simulink model "SPMSM_Speed_Control"  (R2023b)
settings: Solver=ode45  StartTime=0.0  StopTime=10  MaxStep=0.001  RelTol=1e-3
values from neighbouring files (symbols this model uses):
  J_motor = 0.0027    [PMSM_parameter2.m]
  Lamda = 0.1194    [PMSM_parameter2.m]
  Ld = 0.0003752    [PMSM_parameter2.m]
  Lq = 0.0003752    [PMSM_parameter2.m]
  Pole = 2    [PMSM_parameter2.m]
  R = 0.2    [PMSM_parameter2.m]
  T_load = 10    [PMSM_parameter2.m]
  w_base = (60/(2*pi))*(v_rated/sqrt((Ls^2)*(T_load/1.5*Pole*Lamda)^2+(Lamda^2)))    [PMSM_parameter2.m]
  w_ref = 3000    [PMSM_parameter2.m]
undefined symbols (not defined in the file or in its folder): v_rated
libraries: mcbcontrolslib x10, slpidlib x6, autolibpmsmexterior x2, simulink_extras x1, autolibpmsmcommon x1, spsSawtoothGeneratorLib x1
settings Model: Creator=chayutht  LastModifiedBy=chayutht
settings DebuggingCC: AlgebraicLoopMsg=none  ArtificialAlgebraicLoopMsg=none

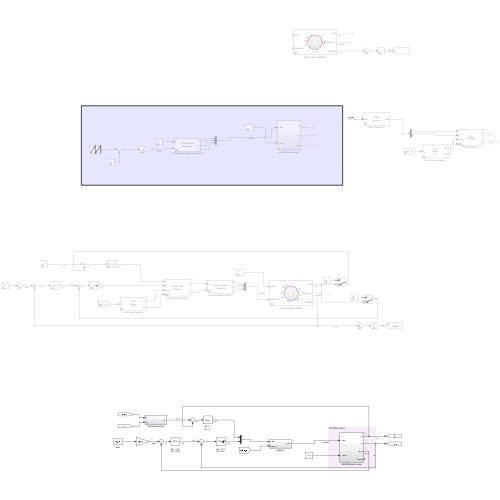
[thumbnail: Simulink's stored preview of the top-level diagram]
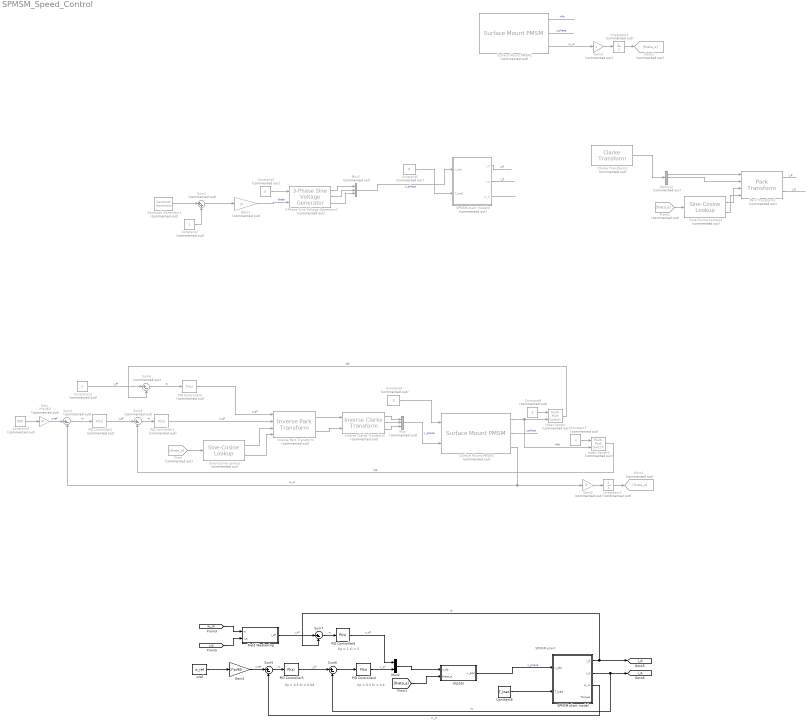
== system SPMSM_Speed_Control ==
  note: SPMSM plant
  note: Kp = 1
      | Ki = 5
  note: Kp = 0.3
      | Ki = 0.4
  note: Kp = 0.5
      | Ki = 0.08
  3-Phase Sine Voltage Generator2 : mcbcontrolslib/3-Phase Sine Voltage Generator  Commented=on  AngleInput=Radians  N_points=1024
      settings: LibrarySourceBlock=mcblib/Controls/Math Transforms/3-Phase Sine Voltage Generator
  Clarke Transform1 : mcbcontrolslib/Clarke Transform  Commented=on  VariantControl=Variant2  PhaseInput=Three inputs  EnPowerInv=off
      settings: LibrarySourceBlock=mcblib/Controls/Math Transforms/Clarke Transform
  Constant10 : Constant  Commented=on  Value=0
  Constant2 : Constant  Commented=on
  Constant3 : Constant  Commented=on  Value=5
  Constant4 : Constant  Commented=on  Value=0
  Constant5 : Constant  Commented=on  Value=0
  Constant6 : Constant  Commented=on  Value=3
  Constant7 : Constant  Commented=on  Value=4
  Constant8 : Constant  Value=T_load
  Constant9 : Constant  Commented=on  Value=500
  Demux2 : Demux  Commented=on  Outputs=3
  Field Weakening : Subsystem
  From : From  Commented=on  GotoTag=theta_e
  From2 : From  Commented=on  GotoTag=theta_e
  Gain : Gain  Commented=on  Gain=2*pi/60
  Gain1 : Gain  Commented=on  Gain=pi
  Gain2 : Gain  Commented=on  Gain=2
  Gain3 : Gain  Commented=on  Gain=2
  Gain4 : Gain  Gain=2*pi/60
  Goto1 : Goto  Commented=on  GotoTag=theta_e
  Goto2 : Goto  Commented=on  GotoTag=theta_e
  Index Vector : MultiPortSwitch  Commented=on  DataPortOrder=Zero-based contiguous  Inputs=1  zeroidx=on  SaturateOnIntegerOverflow=off  InputSameDT=off
  Index Vector1 : MultiPortSwitch  Commented=on  DataPortOrder=Zero-based contiguous  Inputs=1  zeroidx=on  SaturateOnIntegerOverflow=off  InputSameDT=off
  Integrator1 : Integrator  Commented=on
  Integrator2 : Integrator  Commented=on
  Inverse Clarke Transform : mcbcontrolslib/Inverse Clarke Transform  Commented=on  PhaseInput=Two inputs  EnPowerInv=off
      settings: LibrarySourceBlock=mcblib/Controls/Math Transforms/Inverse Clarke Transform
  Inverse Park Transform : mcbcontrolslib/Inverse Park Transform  Commented=on  PhaseInput=Two inputs  AxisAlignment=D-axis  ThetaInput=Sine and Cosine electrical position  AngleInput=Per-unit  N_points=1024
      settings: LibrarySourceBlock=mcblib/Controls/Math Transforms/Inverse Park Transform
  Mux : Mux  Commented=on  Inputs=3
  Mux1 : Mux  Commented=on  Inputs=3
  Mux2 : Mux  Inputs=2
  PID Controller1 : slpidlib/PID Controller  Commented=on  Controller=PI  Form=Parallel  TimeDomain=Continuous-time  UseExternalTs=off  SampleTime=-1  IntegratorMethod=Forward Euler  FilterMethod=Forward Euler  ControllerParametersSource=internal  P=3  I=1  UseKiTs=off  D=0  N=100  UseFilter=on  TunerSelectOption=Transfer Function Based (PID Tuner App)  InitialConditionSource=internal  InitialConditionForIntegrator=0  InitialConditionForFilter=0  DifferentiatorICPrevScaledInput=0  ExternalReset=none  TrackingMode=off  Kt=1  LimitOutput=on  SatLimitsSource=internal  UpperSaturationLimit=200  LowerSaturationLimit=-200  LinearizeAsGain=off  AntiWindupMode=none  Kb=1  LimitIntegrator=off  UpperIntegratorSaturationLimit=inf  LowerIntegratorSaturationLimit=-inf  POutMin=[]  POutMax=[]  IOutMin=[]  IOutMax=[]  DOutMin=[]  DOutMax=[]  NOutMin=[]  NOutMax=[]  SumOutMin=[]  SumOutMax=[]  SaturationOutMin=[]  SaturationOutMax=[]  PParamMin=[]  PParamMax=[]  IParamMin=[]  IParamMax=[]  DParamMin=[]  DParamMax=[]  NParamMin=[]  NParamMax=[]  KbParamMin=[]  KbParamMax=[]  KtParamMin=[]  KtParamMax=[]  KbOutMin=[]  KbOutMax=[]  KtOutMin=[]  KtOutMax=[]  IntegratorOutMin=[]  IntegratorOutMax=[]  FilterOutMin=[]  FilterOutMax=[]  SumI1OutMin=[]  SumI1OutMax=[]  SumI2OutMin=[]  SumI2OutMax=[]  SumI3OutMin=[]  SumI3OutMax=[]  SumI4OutMin=[]  SumI4OutMax=[]  SumDOutMin=[]  SumDOutMax=[]  DifferentiatorOutMin=[]  DifferentiatorOutMax=[]  FilterDiffOutCoefMin=[]  FilterDiffOutCoefMax=[]  ReciprocalOutMin=[]  ReciprocalOutMax=[]  SumDenOutMin=[]  SumDenOutMax=[]  SumNumOutMin=[]  SumNumOutMax=[]  DivideOutMin=[]  DivideOutMax=[]  UdiffTsProdOutMin=[]  UdiffTsProdOutMax=[]  NTsProdOutMin=[]  NTsProdOutMax=[]  UintegralTsProdOutMin=[]  UintegralTsProdOutMax=[]  UngainTsProdOutMin=[]  UngainTsProdOutMax=[]  ClampingZeroOutDataTypeStr=Inherit: Inherit via back propagation  ClampingZeroOutMin=[]  ClampingZeroOutMax=[]  FilterDenConstantOutDataTypeStr=Inherit: Inherit via back propagation  FilterDenConstantOutMin=[]  FilterDenConstantOutMax=[]  PCopyOutDataTypeStr=Inherit: Inherit via back propagation  PCopyOutMin=[]  PCopyOutMax=[]  NCopyOutDataTypeStr=Inherit: Inherit via back propagation  NCopyOutMin=[]  NCopyOutMax=[]  IntegratorContinuousStateAttributes=''  IntegratorStateMustResolveToSignalObject=off  IntegratorRTWStateStorageClass=Auto  FilterContinuousStateAttributes=''  FilterStateMustResolveToSignalObject=off  FilterRTWStateStorageClass=Auto  ParallelPVariant=InternalParameters  IdealPVariant=Disabled  IVariant=InternalParameters  DVariant=Disabled  IntegratorVariant=Continuous  SatVariant=Enabled  AWVariant=Passthrough  PCopyVariant=Disabled  TRVariant=Disabled  FdbkBlocksVariant=Forward  IdealPFdbkVariant=Disabled  SatFdbkVariant=Disabled  DerivativeFilterVariant=Disabled  NVariant=Disabled  NCopyVariant=Disabled_SignalSpec  FilterICVariant=Disabled  IntegratorICVariant=InternalICs  ExternalResetVariant=Disabled  TRSumVariant=Passthrough  SumFdbkVariant=Disabled  SumVariant=Sum_PI  TsampFilterVariant=InternalTs  TsampNgainVariant=Passthrough  TsampIntegralVariant=Disabled_SignalSpec  ExternalSaturationOutDataTypeStr=Inherit: Same as second input
  PID Controller2 : slpidlib/PID Controller  Commented=on  Controller=PI  Form=Parallel  TimeDomain=Continuous-time  UseExternalTs=off  SampleTime=-1  IntegratorMethod=Forward Euler  FilterMethod=Forward Euler  ControllerParametersSource=internal  P=1  I=2  UseKiTs=off  D=0  N=100  UseFilter=on  TunerSelectOption=Transfer Function Based (PID Tuner App)  InitialConditionSource=internal  InitialConditionForIntegrator=0  InitialConditionForFilter=0  DifferentiatorICPrevScaledInput=0  ExternalReset=none  TrackingMode=off  Kt=1  LimitOutput=off  SatLimitsSource=internal  UpperSaturationLimit=inf  LowerSaturationLimit=-inf  LinearizeAsGain=on  AntiWindupMode=none  Kb=1  LimitIntegrator=off  UpperIntegratorSaturationLimit=inf  LowerIntegratorSaturationLimit=-inf  POutMin=[]  POutMax=[]  IOutMin=[]  IOutMax=[]  DOutMin=[]  DOutMax=[]  NOutMin=[]  NOutMax=[]  SumOutMin=[]  SumOutMax=[]  SaturationOutMin=[]  SaturationOutMax=[]  PParamMin=[]  PParamMax=[]  IParamMin=[]  IParamMax=[]  DParamMin=[]  DParamMax=[]  NParamMin=[]  NParamMax=[]  KbParamMin=[]  KbParamMax=[]  KtParamMin=[]  KtParamMax=[]  KbOutMin=[]  KbOutMax=[]  KtOutMin=[]  KtOutMax=[]  IntegratorOutMin=[]  IntegratorOutMax=[]  FilterOutMin=[]  FilterOutMax=[]  SumI1OutMin=[]  SumI1OutMax=[]  SumI2OutMin=[]  SumI2OutMax=[]  SumI3OutMin=[]  SumI3OutMax=[]  SumI4OutMin=[]  SumI4OutMax=[]  SumDOutMin=[]  SumDOutMax=[]  DifferentiatorOutMin=[]  DifferentiatorOutMax=[]  FilterDiffOutCoefMin=[]  FilterDiffOutCoefMax=[]  ReciprocalOutMin=[]  ReciprocalOutMax=[]  SumDenOutMin=[]  SumDenOutMax=[]  SumNumOutMin=[]  SumNumOutMax=[]  DivideOutMin=[]  DivideOutMax=[]  UdiffTsProdOutMin=[]  UdiffTsProdOutMax=[]  NTsProdOutMin=[]  NTsProdOutMax=[]  UintegralTsProdOutMin=[]  UintegralTsProdOutMax=[]  UngainTsProdOutMin=[]  UngainTsProdOutMax=[]  ClampingZeroOutDataTypeStr=Inherit: Inherit via back propagation  ClampingZeroOutMin=[]  ClampingZeroOutMax=[]  FilterDenConstantOutDataTypeStr=Inherit: Inherit via back propagation  FilterDenConstantOutMin=[]  FilterDenConstantOutMax=[]  PCopyOutDataTypeStr=Inherit: Inherit via back propagation  PCopyOutMin=[]  PCopyOutMax=[]  NCopyOutDataTypeStr=Inherit: Inherit via back propagation  NCopyOutMin=[]  NCopyOutMax=[]  IntegratorContinuousStateAttributes=''  IntegratorStateMustResolveToSignalObject=off  IntegratorRTWStateStorageClass=Auto  FilterContinuousStateAttributes=''  FilterStateMustResolveToSignalObject=off  FilterRTWStateStorageClass=Auto  ParallelPVariant=InternalParameters  IdealPVariant=Disabled  IVariant=InternalParameters  DVariant=Disabled  IntegratorVariant=Continuous  SatVariant=Disabled  AWVariant=Passthrough  PCopyVariant=Disabled  TRVariant=Disabled  FdbkBlocksVariant=Forward  IdealPFdbkVariant=Disabled  SatFdbkVariant=Disabled  DerivativeFilterVariant=Disabled  NVariant=Disabled  NCopyVariant=Disabled_SignalSpec  FilterICVariant=Disabled  IntegratorICVariant=InternalICs  ExternalResetVariant=Disabled  TRSumVariant=Passthrough  SumFdbkVariant=Disabled  SumVariant=Sum_PI  TsampFilterVariant=InternalTs  TsampNgainVariant=Passthrough  TsampIntegralVariant=Disabled_SignalSpec  ExternalSaturationOutDataTypeStr=Inherit: Same as second input
  PID Controller3 : slpidlib/PID Controller  Commented=on  Controller=PI  Form=Parallel  TimeDomain=Continuous-time  UseExternalTs=off  SampleTime=-1  IntegratorMethod=Forward Euler  FilterMethod=Forward Euler  ControllerParametersSource=internal  P=0.5  I=1  UseKiTs=off  D=0  N=100  UseFilter=on  TunerSelectOption=Transfer Function Based (PID Tuner App)  InitialConditionSource=internal  InitialConditionForIntegrator=0  InitialConditionForFilter=0  DifferentiatorICPrevScaledInput=0  ExternalReset=none  TrackingMode=off  Kt=1  LimitOutput=off  SatLimitsSource=internal  UpperSaturationLimit=inf  LowerSaturationLimit=-inf  LinearizeAsGain=on  AntiWindupMode=none  Kb=1  LimitIntegrator=off  UpperIntegratorSaturationLimit=inf  LowerIntegratorSaturationLimit=-inf  POutMin=[]  POutMax=[]  IOutMin=[]  IOutMax=[]  DOutMin=[]  DOutMax=[]  NOutMin=[]  NOutMax=[]  SumOutMin=[]  SumOutMax=[]  SaturationOutMin=[]  SaturationOutMax=[]  PParamMin=[]  PParamMax=[]  IParamMin=[]  IParamMax=[]  DParamMin=[]  DParamMax=[]  NParamMin=[]  NParamMax=[]  KbParamMin=[]  KbParamMax=[]  KtParamMin=[]  KtParamMax=[]  KbOutMin=[]  KbOutMax=[]  KtOutMin=[]  KtOutMax=[]  IntegratorOutMin=[]  IntegratorOutMax=[]  FilterOutMin=[]  FilterOutMax=[]  SumI1OutMin=[]  SumI1OutMax=[]  SumI2OutMin=[]  SumI2OutMax=[]  SumI3OutMin=[]  SumI3OutMax=[]  SumI4OutMin=[]  SumI4OutMax=[]  SumDOutMin=[]  SumDOutMax=[]  DifferentiatorOutMin=[]  DifferentiatorOutMax=[]  FilterDiffOutCoefMin=[]  FilterDiffOutCoefMax=[]  ReciprocalOutMin=[]  ReciprocalOutMax=[]  SumDenOutMin=[]  SumDenOutMax=[]  SumNumOutMin=[]  SumNumOutMax=[]  DivideOutMin=[]  DivideOutMax=[]  UdiffTsProdOutMin=[]  UdiffTsProdOutMax=[]  NTsProdOutMin=[]  NTsProdOutMax=[]  UintegralTsProdOutMin=[]  UintegralTsProdOutMax=[]  UngainTsProdOutMin=[]  UngainTsProdOutMax=[]  ClampingZeroOutDataTypeStr=Inherit: Inherit via back propagation  ClampingZeroOutMin=[]  ClampingZeroOutMax=[]  FilterDenConstantOutDataTypeStr=Inherit: Inherit via back propagation  FilterDenConstantOutMin=[]  FilterDenConstantOutMax=[]  PCopyOutDataTypeStr=Inherit: Inherit via back propagation  PCopyOutMin=[]  PCopyOutMax=[]  NCopyOutDataTypeStr=Inherit: Inherit via back propagation  NCopyOutMin=[]  NCopyOutMax=[]  IntegratorContinuousStateAttributes=''  IntegratorStateMustResolveToSignalObject=off  IntegratorRTWStateStorageClass=Auto  FilterContinuousStateAttributes=''  FilterStateMustResolveToSignalObject=off  FilterRTWStateStorageClass=Auto  ParallelPVariant=InternalParameters  IdealPVariant=Disabled  IVariant=InternalParameters  DVariant=Disabled  IntegratorVariant=Continuous  SatVariant=Disabled  AWVariant=Passthrough  PCopyVariant=Disabled  TRVariant=Disabled  FdbkBlocksVariant=Forward  IdealPFdbkVariant=Disabled  SatFdbkVariant=Disabled  DerivativeFilterVariant=Disabled  NVariant=Disabled  NCopyVariant=Disabled_SignalSpec  FilterICVariant=Disabled  IntegratorICVariant=InternalICs  ExternalResetVariant=Disabled  TRSumVariant=Passthrough  SumFdbkVariant=Disabled  SumVariant=Sum_PI  TsampFilterVariant=InternalTs  TsampNgainVariant=Passthrough  TsampIntegralVariant=Disabled_SignalSpec  ExternalSaturationOutDataTypeStr=Inherit: Same as second input
  PID Controller4 : slpidlib/PID Controller  Controller=PI  Form=Parallel  TimeDomain=Continuous-time  UseExternalTs=off  SampleTime=-1  IntegratorMethod=Forward Euler  FilterMethod=Forward Euler  ControllerParametersSource=internal  P=0.3  I=0.4  UseKiTs=off  D=0  N=100  UseFilter=on  TunerSelectOption=Transfer Function Based (PID Tuner App)  InitialConditionSource=internal  InitialConditionForIntegrator=0  InitialConditionForFilter=0  DifferentiatorICPrevScaledInput=0  ExternalReset=none  TrackingMode=off  Kt=1  LimitOutput=on  SatLimitsSource=internal  UpperSaturationLimit=200  LowerSaturationLimit=-200  LinearizeAsGain=off  AntiWindupMode=none  Kb=1  LimitIntegrator=off  UpperIntegratorSaturationLimit=inf  LowerIntegratorSaturationLimit=-inf  POutMin=[]  POutMax=[]  IOutMin=[]  IOutMax=[]  DOutMin=[]  DOutMax=[]  NOutMin=[]  NOutMax=[]  SumOutMin=[]  SumOutMax=[]  SaturationOutMin=[]  SaturationOutMax=[]  PParamMin=[]  PParamMax=[]  IParamMin=[]  IParamMax=[]  DParamMin=[]  DParamMax=[]  NParamMin=[]  NParamMax=[]  KbParamMin=[]  KbParamMax=[]  KtParamMin=[]  KtParamMax=[]  KbOutMin=[]  KbOutMax=[]  KtOutMin=[]  KtOutMax=[]  IntegratorOutMin=[]  IntegratorOutMax=[]  FilterOutMin=[]  FilterOutMax=[]  SumI1OutMin=[]  SumI1OutMax=[]  SumI2OutMin=[]  SumI2OutMax=[]  SumI3OutMin=[]  SumI3OutMax=[]  SumI4OutMin=[]  SumI4OutMax=[]  SumDOutMin=[]  SumDOutMax=[]  DifferentiatorOutMin=[]  DifferentiatorOutMax=[]  FilterDiffOutCoefMin=[]  FilterDiffOutCoefMax=[]  ReciprocalOutMin=[]  ReciprocalOutMax=[]  SumDenOutMin=[]  SumDenOutMax=[]  SumNumOutMin=[]  SumNumOutMax=[]  DivideOutMin=[]  DivideOutMax=[]  UdiffTsProdOutMin=[]  UdiffTsProdOutMax=[]  NTsProdOutMin=[]  NTsProdOutMax=[]  UintegralTsProdOutMin=[]  UintegralTsProdOutMax=[]  UngainTsProdOutMin=[]  UngainTsProdOutMax=[]  ClampingZeroOutDataTypeStr=Inherit: Inherit via back propagation  ClampingZeroOutMin=[]  ClampingZeroOutMax=[]  FilterDenConstantOutDataTypeStr=Inherit: Inherit via back propagation  FilterDenConstantOutMin=[]  FilterDenConstantOutMax=[]  PCopyOutDataTypeStr=Inherit: Inherit via back propagation  PCopyOutMin=[]  PCopyOutMax=[]  NCopyOutDataTypeStr=Inherit: Inherit via back propagation  NCopyOutMin=[]  NCopyOutMax=[]  IntegratorContinuousStateAttributes=''  IntegratorStateMustResolveToSignalObject=off  IntegratorRTWStateStorageClass=Auto  FilterContinuousStateAttributes=''  FilterStateMustResolveToSignalObject=off  FilterRTWStateStorageClass=Auto  ParallelPVariant=InternalParameters  IdealPVariant=Disabled  IVariant=InternalParameters  DVariant=Disabled  IntegratorVariant=Continuous  SatVariant=Enabled  AWVariant=Passthrough  PCopyVariant=Disabled  TRVariant=Disabled  FdbkBlocksVariant=Forward  IdealPFdbkVariant=Disabled  SatFdbkVariant=Disabled  DerivativeFilterVariant=Disabled  NVariant=Disabled  NCopyVariant=Disabled_SignalSpec  FilterICVariant=Disabled  IntegratorICVariant=InternalICs  ExternalResetVariant=Disabled  TRSumVariant=Passthrough  SumFdbkVariant=Disabled  SumVariant=Sum_PI  TsampFilterVariant=InternalTs  TsampNgainVariant=Passthrough  TsampIntegralVariant=Disabled_SignalSpec  ExternalSaturationOutDataTypeStr=Inherit: Same as second input
  PID Controller5 : slpidlib/PID Controller  Controller=PI  Form=Parallel  TimeDomain=Continuous-time  UseExternalTs=off  SampleTime=-1  IntegratorMethod=Forward Euler  FilterMethod=Forward Euler  ControllerParametersSource=internal  P=0.5  I=0.08  UseKiTs=off  D=0  N=100  UseFilter=on  TunerSelectOption=Transfer Function Based (PID Tuner App)  InitialConditionSource=internal  InitialConditionForIntegrator=0  InitialConditionForFilter=0  DifferentiatorICPrevScaledInput=0  ExternalReset=none  TrackingMode=off  Kt=1  LimitOutput=off  SatLimitsSource=internal  UpperSaturationLimit=inf  LowerSaturationLimit=-inf  LinearizeAsGain=on  AntiWindupMode=none  Kb=1  LimitIntegrator=off  UpperIntegratorSaturationLimit=inf  LowerIntegratorSaturationLimit=-inf  POutMin=[]  POutMax=[]  IOutMin=[]  IOutMax=[]  DOutMin=[]  DOutMax=[]  NOutMin=[]  NOutMax=[]  SumOutMin=[]  SumOutMax=[]  SaturationOutMin=[]  SaturationOutMax=[]  PParamMin=[]  PParamMax=[]  IParamMin=[]  IParamMax=[]  DParamMin=[]  DParamMax=[]  NParamMin=[]  NParamMax=[]  KbParamMin=[]  KbParamMax=[]  KtParamMin=[]  KtParamMax=[]  KbOutMin=[]  KbOutMax=[]  KtOutMin=[]  KtOutMax=[]  IntegratorOutMin=[]  IntegratorOutMax=[]  FilterOutMin=[]  FilterOutMax=[]  SumI1OutMin=[]  SumI1OutMax=[]  SumI2OutMin=[]  SumI2OutMax=[]  SumI3OutMin=[]  SumI3OutMax=[]  SumI4OutMin=[]  SumI4OutMax=[]  SumDOutMin=[]  SumDOutMax=[]  DifferentiatorOutMin=[]  DifferentiatorOutMax=[]  FilterDiffOutCoefMin=[]  FilterDiffOutCoefMax=[]  ReciprocalOutMin=[]  ReciprocalOutMax=[]  SumDenOutMin=[]  SumDenOutMax=[]  SumNumOutMin=[]  SumNumOutMax=[]  DivideOutMin=[]  DivideOutMax=[]  UdiffTsProdOutMin=[]  UdiffTsProdOutMax=[]  NTsProdOutMin=[]  NTsProdOutMax=[]  UintegralTsProdOutMin=[]  UintegralTsProdOutMax=[]  UngainTsProdOutMin=[]  UngainTsProdOutMax=[]  ClampingZeroOutDataTypeStr=Inherit: Inherit via back propagation  ClampingZeroOutMin=[]  ClampingZeroOutMax=[]  FilterDenConstantOutDataTypeStr=Inherit: Inherit via back propagation  FilterDenConstantOutMin=[]  FilterDenConstantOutMax=[]  PCopyOutDataTypeStr=Inherit: Inherit via back propagation  PCopyOutMin=[]  PCopyOutMax=[]  NCopyOutDataTypeStr=Inherit: Inherit via back propagation  NCopyOutMin=[]  NCopyOutMax=[]  IntegratorContinuousStateAttributes=''  IntegratorStateMustResolveToSignalObject=off  IntegratorRTWStateStorageClass=Auto  FilterContinuousStateAttributes=''  FilterStateMustResolveToSignalObject=off  FilterRTWStateStorageClass=Auto  ParallelPVariant=InternalParameters  IdealPVariant=Disabled  IVariant=InternalParameters  DVariant=Disabled  IntegratorVariant=Continuous  SatVariant=Disabled  AWVariant=Passthrough  PCopyVariant=Disabled  TRVariant=Disabled  FdbkBlocksVariant=Forward  IdealPFdbkVariant=Disabled  SatFdbkVariant=Disabled  DerivativeFilterVariant=Disabled  NVariant=Disabled  NCopyVariant=Disabled_SignalSpec  FilterICVariant=Disabled  IntegratorICVariant=InternalICs  ExternalResetVariant=Disabled  TRSumVariant=Passthrough  SumFdbkVariant=Disabled  SumVariant=Sum_PI  TsampFilterVariant=InternalTs  TsampNgainVariant=Passthrough  TsampIntegralVariant=Disabled_SignalSpec  ExternalSaturationOutDataTypeStr=Inherit: Same as second input
  PID Controller6 : slpidlib/PID Controller  Controller=PI  Form=Parallel  TimeDomain=Continuous-time  UseExternalTs=off  SampleTime=-1  IntegratorMethod=Forward Euler  FilterMethod=Forward Euler  ControllerParametersSource=internal  P=1  I=5  UseKiTs=off  D=0  N=100  UseFilter=on  TunerSelectOption=Transfer Function Based (PID Tuner App)  InitialConditionSource=internal  InitialConditionForIntegrator=0  InitialConditionForFilter=0  DifferentiatorICPrevScaledInput=0  ExternalReset=none  TrackingMode=off  Kt=1  LimitOutput=off  SatLimitsSource=internal  UpperSaturationLimit=inf  LowerSaturationLimit=-inf  LinearizeAsGain=on  AntiWindupMode=none  Kb=1  LimitIntegrator=off  UpperIntegratorSaturationLimit=inf  LowerIntegratorSaturationLimit=-inf  POutMin=[]  POutMax=[]  IOutMin=[]  IOutMax=[]  DOutMin=[]  DOutMax=[]  NOutMin=[]  NOutMax=[]  SumOutMin=[]  SumOutMax=[]  SaturationOutMin=[]  SaturationOutMax=[]  PParamMin=[]  PParamMax=[]  IParamMin=[]  IParamMax=[]  DParamMin=[]  DParamMax=[]  NParamMin=[]  NParamMax=[]  KbParamMin=[]  KbParamMax=[]  KtParamMin=[]  KtParamMax=[]  KbOutMin=[]  KbOutMax=[]  KtOutMin=[]  KtOutMax=[]  IntegratorOutMin=[]  IntegratorOutMax=[]  FilterOutMin=[]  FilterOutMax=[]  SumI1OutMin=[]  SumI1OutMax=[]  SumI2OutMin=[]  SumI2OutMax=[]  SumI3OutMin=[]  SumI3OutMax=[]  SumI4OutMin=[]  SumI4OutMax=[]  SumDOutMin=[]  SumDOutMax=[]  DifferentiatorOutMin=[]  DifferentiatorOutMax=[]  FilterDiffOutCoefMin=[]  FilterDiffOutCoefMax=[]  ReciprocalOutMin=[]  ReciprocalOutMax=[]  SumDenOutMin=[]  SumDenOutMax=[]  SumNumOutMin=[]  SumNumOutMax=[]  DivideOutMin=[]  DivideOutMax=[]  UdiffTsProdOutMin=[]  UdiffTsProdOutMax=[]  NTsProdOutMin=[]  NTsProdOutMax=[]  UintegralTsProdOutMin=[]  UintegralTsProdOutMax=[]  UngainTsProdOutMin=[]  UngainTsProdOutMax=[]  ClampingZeroOutDataTypeStr=Inherit: Inherit via back propagation  ClampingZeroOutMin=[]  ClampingZeroOutMax=[]  FilterDenConstantOutDataTypeStr=Inherit: Inherit via back propagation  FilterDenConstantOutMin=[]  FilterDenConstantOutMax=[]  PCopyOutDataTypeStr=Inherit: Inherit via back propagation  PCopyOutMin=[]  PCopyOutMax=[]  NCopyOutDataTypeStr=Inherit: Inherit via back propagation  NCopyOutMin=[]  NCopyOutMax=[]  IntegratorContinuousStateAttributes=''  IntegratorStateMustResolveToSignalObject=off  IntegratorRTWStateStorageClass=Auto  FilterContinuousStateAttributes=''  FilterStateMustResolveToSignalObject=off  FilterRTWStateStorageClass=Auto  ParallelPVariant=InternalParameters  IdealPVariant=Disabled  IVariant=InternalParameters  DVariant=Disabled  IntegratorVariant=Continuous  SatVariant=Disabled  AWVariant=Passthrough  PCopyVariant=Disabled  TRVariant=Disabled  FdbkBlocksVariant=Forward  IdealPFdbkVariant=Disabled  SatFdbkVariant=Disabled  DerivativeFilterVariant=Disabled  NVariant=Disabled  NCopyVariant=Disabled_SignalSpec  FilterICVariant=Disabled  IntegratorICVariant=InternalICs  ExternalResetVariant=Disabled  TRSumVariant=Passthrough  SumFdbkVariant=Disabled  SumVariant=Sum_PI  TsampFilterVariant=InternalTs  TsampNgainVariant=Passthrough  TsampIntegralVariant=Disabled_SignalSpec  ExternalSaturationOutDataTypeStr=Inherit: Same as second input
  Park Transform1 : mcbcontrolslib/Park Transform  Commented=on  PhaseInput=Two inputs  AxisAlignment=D-axis  ThetaInput=Sine and Cosine electrical position  AngleInput=Per-unit  N_points=1024
      settings: LibrarySourceBlock=mcblib/Controls/Math Transforms/Park Transform
  SPMSM plant model : Subsystem
  SPMSM plant model0 : Subsystem  Commented=on
  Sawtooth Generator1 : spsSawtoothGeneratorLib/Sawtooth Generator  Commented=on  Freq=1  Phase=0  Ts=0
  Sine-Cosine Lookup : mcbcontrolslib/Sine-Cosine Lookup  Commented=on  AngleInput=Radians  N_points=1024
      settings: LibrarySourceBlock=mcblib/Controls/Math Transforms/Sine-Cosine Lookup
  Sine-Cosine Lookup2 : mcbcontrolslib/Sine-Cosine Lookup  Commented=on  AngleInput=Radians  N_points=1024
      settings: LibrarySourceBlock=mcblib/Controls/Math Transforms/Sine-Cosine Lookup
  Sum1 : Sum  Commented=on  Inputs=|++
  Sum2 : Sum  Commented=on  Inputs=|+-
  Sum3 : Sum  Commented=on  Inputs=|+-
  Sum4 : Sum  Commented=on  Inputs=|+-
  Sum5 : Sum  Inputs=|+-
  Sum6 : Sum  Inputs=|+-
  Sum7 : Sum  Inputs=|+-
  Surface Mount PMSM1 : autolibpmsmexterior/Surface Mount PMSM  Commented=on  port_config=Torque  sim_type=Continuous  Ts=0.001  FilePath=E:\Sandbox\Bauto\Work\surfacepmsm_motordata.m  P=2  Rs=.2  Ldq_=3.752e-4  KConstText=Permanent flux linkage constant (lambda_pm):  lambda_pm=0.1194  Ke=159.9771  Kt=1.323  mechanical=[0.0027, 4.924e-4, 0]  idq0=[0 0]  theta_init=0  omega_init=0  KConst=0.1194  lambda_pm_calc=0.1194  RefBlkName='autolibpmsmexterior/Surface Mount PMSM'  aMode=1  Ldq="[0.0003752   0.0003752]"
      settings: LibrarySourceBlock=autolibemachines/Surface Mount PMSM
  Surface Mount PMSM2 : autolibpmsmexterior/Surface Mount PMSM  Commented=on  port_config=Torque  sim_type=Continuous  Ts=0.001  FilePath=E:\Sandbox\Bauto\Work\surfacepmsm_motordata.m  P=2  Rs=.2  Ldq_=3.752e-4  KConstText=Permanent flux linkage constant (lambda_pm):  lambda_pm=0.1194  Ke=159.9771  Kt=1.323  mechanical=[0.0027, 4.924e-4, 0]  idq0=[0 0]  theta_init=0  omega_init=0  KConst=0.1194  lambda_pm_calc=0.1194  RefBlkName='autolibpmsmexterior/Surface Mount PMSM'  aMode=1  Ldq="[0.0003752   0.0003752]"
      settings: LibrarySourceBlock=autolibemachines/Surface Mount PMSM
  dq2abc : Subsystem
  wref : Constant  Value=w_ref
  tag scope: i_d=global, i_q=global
  wires:
  Constant4/1 -> Surface Mount PMSM2/1
  Mux/1 -> Surface Mount PMSM2/2  "v_phase"
  Gain1/1 -> 3-Phase Sine Voltage Generator2/2  "theta"
  Sawtooth Generator1/1 -> Sum1/1
  Constant3/1 -> 3-Phase Sine Voltage Generator2/1
  Constant2/1 -> Sum1/2
  3-Phase Sine Voltage Generator2/1 -> Mux1/1
  3-Phase Sine Voltage Generator2/3 -> Mux1/3
  Sum1/1 -> Gain1/1
  Mux1/1 -> SPMSM plant model0/1(v_abc)  "v_phase"
  3-Phase Sine Voltage Generator2/2 -> Mux1/2
  Constant5/1 -> SPMSM plant model0/2(T_load)
  Inverse Clarke Transform/2 -> Mux/2
  Inverse Clarke Transform/3 -> Mux/3
  Inverse Clarke Transform/1 -> Mux/1
  Inverse Park Transform/1 -> Inverse Clarke Transform/1
  Inverse Park Transform/2 -> Inverse Clarke Transform/2
  Sine-Cosine Lookup/1 -> Inverse Park Transform/3
  Sine-Cosine Lookup/2 -> Inverse Park Transform/4
  ? -> Clarke Transform1/1  "i_phase"
  Demux2/1 -> Park Transform1/1
  Park Transform1/2 -> ?  "i_q"
  Demux2/2 -> Park Transform1/2
  Sine-Cosine Lookup2/1 -> Park Transform1/3
  Sine-Cosine Lookup2/2 -> Park Transform1/4
  Park Transform1/1 -> ?  "i_d"
  From2/1 -> Sine-Cosine Lookup2/1
  Clarke Transform1/1 -> Demux2/1
  SPMSM plant model0/1(i_d) -> ?  "i_d."
  SPMSM plant model0/2(i_q) -> ?  "i_q."
  Surface Mount PMSM1/3 -> Gain2/1  "w_m"
  Gain2/1 -> Integrator1/1
  Integrator1/1 -> Goto2/1
  SPMSM plant model0/3(w_m) -> ?
  Surface Mount PMSM1/2 -> ?  "i_phase"
  Surface Mount PMSM1/1 -> ?  "info"
  From/1 -> Sine-Cosine Lookup/1
  PID Controller2/1 -> Sum3/1  "i_q*"
  Sum2/1 -> PID Controller2/1  "w"
  Surface Mount PMSM2/1 -> Index Vector1/2, Index Vector/2  "info"
  Constant6/1 -> Index Vector/1
  Index Vector/1 -> Sum4/2  "idd"
  Index Vector1/1 -> Sum3/2  "iqq"
  Constant7/1 -> Index Vector1/1
  Surface Mount PMSM2/3 -> Gain3/1, Sum2/2  "w_m"
  Integrator2/1 -> Goto1/1
  Gain3/1 -> Integrator2/1
  Surface Mount PMSM2/2 -> ?  "i_phase"
  Constant10/1 -> Sum4/1  "i_d*"
  Constant9/1 -> Gain/1
  Gain/1 -> Sum2/1  "wref"
  PID Controller1/1 -> Inverse Park Transform/2  "v_q*"
  Sum3/1 -> PID Controller1/1  "w"
  Sum4/1 -> PID Controller3/1  "w"
  PID Controller3/1 -> Inverse Park Transform/1  "v_q*"
  Field Weakening/1(i_d*) -> Sum7/1  "i_d*"
  SPMSM plant model/2(i_q) -> Sum6/2, [i_q]  "iq"
  Sum6/1 -> PID Controller4/1
  SPMSM plant model/3(w_m) -> Sum5/2  "w_m"
  wref/1 -> Gain4/1
  [theta_e] -> dq2abc/2(theta_e)
  PID Controller6/1 -> Mux2/1  "v_d*"
  PID Controller5/1 -> Sum6/1  "i_q*"
  PID Controller4/1 -> Mux2/2  "v_q*"
  Sum5/1 -> PID Controller5/1  "w"
  dq2abc/1(v_abc) -> SPMSM plant model/1(v_abc)  "v_phase"
  Constant8/1 -> SPMSM plant model/2(T_load)
  Gain4/1 -> Sum5/1  "wref"
  SPMSM plant model/1(i_d) -> [i_d], Sum7/2  "id"
  Sum7/1 -> PID Controller6/1  "w"
  Mux2/1 -> dq2abc/1(v_dq)
  [w_m] -> Field Weakening/1(w)
  [i_q] -> Field Weakening/2(i_q)

== system SPMSM_Speed_Control/Field Weakening ==
  note: Field Control
  note: state switching condition
  note: constant torque
  w : Inport
  i_q : Inport  Port=2
  Cast To Boolean : DataTypeConversion  OutDataTypeStr=boolean  SaturateOnIntegerOverflow=off  RndMeth=Floor
  Constant : Constant  Value=w_base*2*pi/60
  Constant1 : Constant  Value=0
  Constant2 : Constant  Value=0
  LessThanOrEqual : RelationalOperator  Operator=<=  OutDataTypeStr=boolean  RndMeth=Simplest  InputSameDT=off
  S-R Flip-Flop : simulink_extras/Flip Flops/S-R Flip-Flop  initial_condition=0
  Switch : Switch  Criteria=u2 > Threshold  Threshold=0.5  SaturateOnIntegerOverflow=off  InputSameDT=off
  i_d_control : Subsystem
  i_d* : Outport
  wires:
  Constant/1 -> LessThanOrEqual/1
  LessThanOrEqual/1 -> i_d_control/Enable, S-R Flip-Flop/1  "enable"
  w/1 -> LessThanOrEqual/2, i_d_control/2(w)
  S-R Flip-Flop/1 -> Switch/2
  Constant1/1 -> Switch/3
  Constant2/1 -> Cast To Boolean/1
  Switch/1 -> i_d*/1
  i_q/1 -> i_d_control/1(i_q)
  i_d_control/1(i_d) -> Switch/1
  Cast To Boolean/1 -> S-R Flip-Flop/2

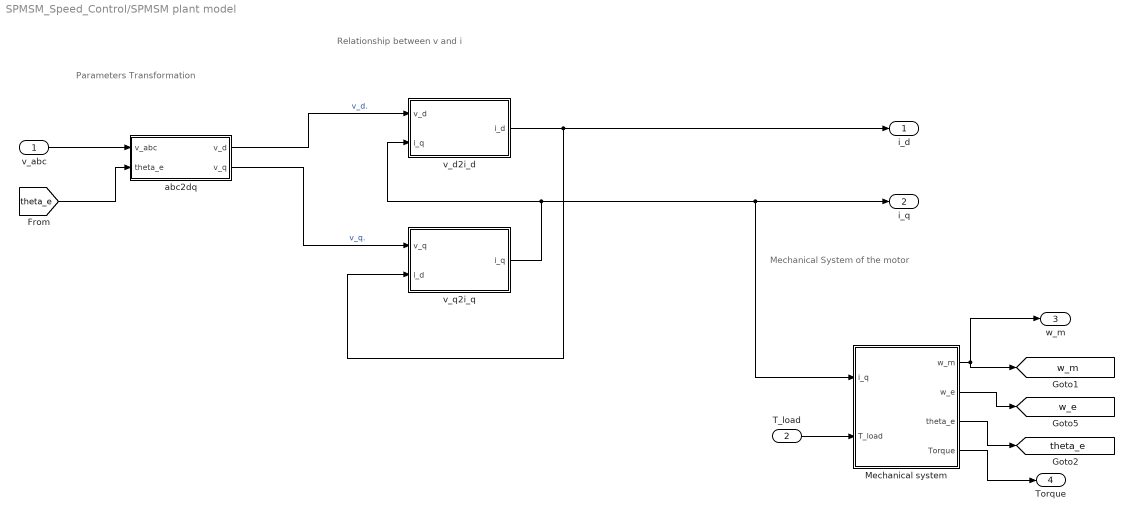
== system SPMSM_Speed_Control/SPMSM plant model ==
  note: Mechanical System of the motor
  note: Relationship between v and i
  note: Parameters Transformation
  v_abc : Inport
  T_load : Inport  Port=2
  Mechanical system : Subsystem
  abc2dq : Subsystem
  v_d2i_d : Subsystem
  v_q2i_q : Subsystem
  i_d : Outport
  i_q : Outport  Port=2
  w_m : Outport  Port=3
  Torque : Outport  Port=4
  tag scope: theta_e=global, w_e=global, w_m=global
  wires:
  v_abc/1 -> abc2dq/1(v_abc)
  abc2dq/2(v_q) -> v_q2i_q/1(v_q)  "v_q."
  [theta_e] -> abc2dq/2(theta_e)
  T_load/1 -> Mechanical system/2(T_load)
  abc2dq/1(v_d) -> v_d2i_d/1(v_d)  "v_d."
  v_d2i_d/1(i_d) -> v_q2i_q/2(i_d), i_d/1
  v_q2i_q/1(i_q) -> v_d2i_d/2(i_q), i_q/1, Mechanical system/1(i_q)
  Mechanical system/1(w_m) -> [w_m], w_m/1
  Mechanical system/3(theta_e) -> [theta_e]
  Mechanical system/2(w_e) -> [w_e]
  Mechanical system/4(Torque) -> Torque/1

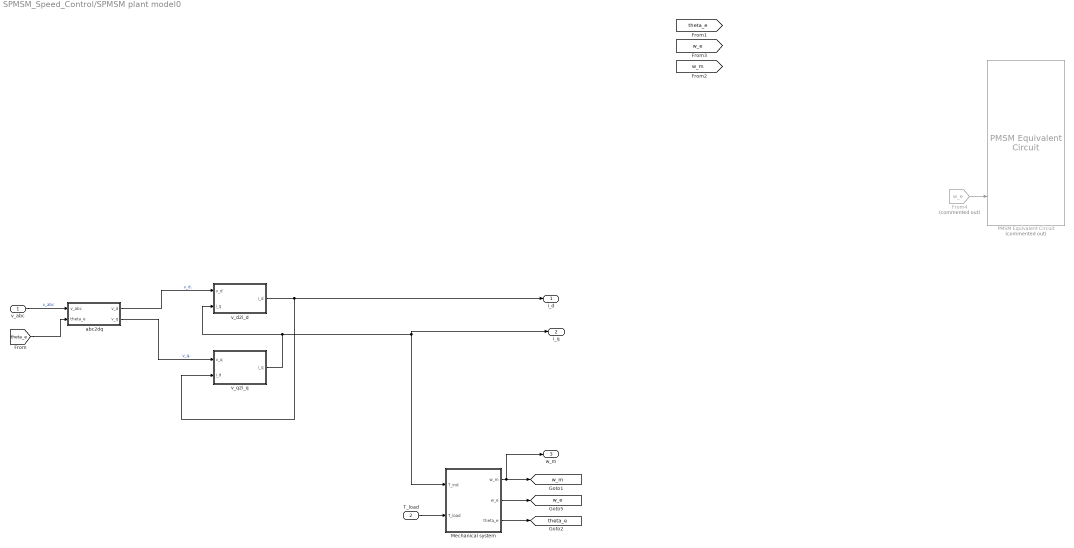
== system SPMSM_Speed_Control/SPMSM plant model0 ==
  v_abc : Inport
  T_load : Inport  Port=2
  From4 : From  Commented=on  GotoTag=w_e  TagVisibility=global
  Mechanical system : Subsystem
  PMSM Equivalent Circuit : autolibpmsmcommon/PMSM Torque Input Core/PMSM Electromagnetic/PMSM Equivalent Circuit  Commented=on  SystemSampleTime=-1  VariantActivationTime=update diagram  AllowFlexibleInterface=on  Latency=0  AutoFrameSizeCalculation=off
  abc2dq : Subsystem
  v_d2i_d : Subsystem
  v_q2i_q : Subsystem
  i_d : Outport
  i_q : Outport  Port=2
  w_m : Outport  Port=3
  tag scope: theta_e=global, w_e=global, w_m=global
  wires:
  v_abc/1 -> abc2dq/1(v_abc)  "v_abc"
  abc2dq/2(v_q) -> v_q2i_q/1(v_q)  "v_q."
  [theta_e] -> abc2dq/2(theta_e)
  T_load/1 -> Mechanical system/2(T_load)
  abc2dq/1(v_d) -> v_d2i_d/1(v_d)  "v_d."
  v_d2i_d/1(i_d) -> i_d/1, v_q2i_q/2(i_d)
  v_q2i_q/1(i_q) -> Mechanical system/1(T_ind), i_q/1, v_d2i_d/2(i_q)
  From4/1 -> PMSM Equivalent Circuit/3
  Mechanical system/1(w_m) -> w_m/1, [w_m]
  Mechanical system/3(theta_e) -> [theta_e]
  Mechanical system/2(w_e) -> [w_e]

== system SPMSM_Speed_Control/dq2abc ==
  note: Inverse Park Transform
  note: Inverse Clark Transform
  v_dq : Inport
  theta_e : Inport  Port=2
  Demux : Demux  Outputs=2
  Mux : Mux  Inputs=3
  Sine-Cosine Lookup1 : mcbcontrolslib/Sine-Cosine Lookup  AngleInput=Radians  N_points=1024
      settings: LibrarySourceBlock=mcblib/Controls/Math Transforms/Sine-Cosine Lookup
  dq2xy : Subsystem
  xy2abc : Subsystem
  v_abc : Outport
  wires:
  theta_e/1 -> Sine-Cosine Lookup1/1
  Sine-Cosine Lookup1/1 -> dq2xy/3(sin_theta)  "sin"
  Sine-Cosine Lookup1/2 -> dq2xy/4(cos_theta)  "cos"
  v_dq/1 -> Demux/1
  Demux/1 -> dq2xy/1(v_d)  "v_d"
  Demux/2 -> dq2xy/2(v_q)  "v_q"
  dq2xy/1(v_xy) -> xy2abc/1(v_xy)  "v_x"
  xy2abc/2(v_b) -> Mux/2
  xy2abc/3(v_c) -> Mux/3
  xy2abc/1(v_a) -> Mux/1
  Mux/1 -> v_abc/1  "v_abc"

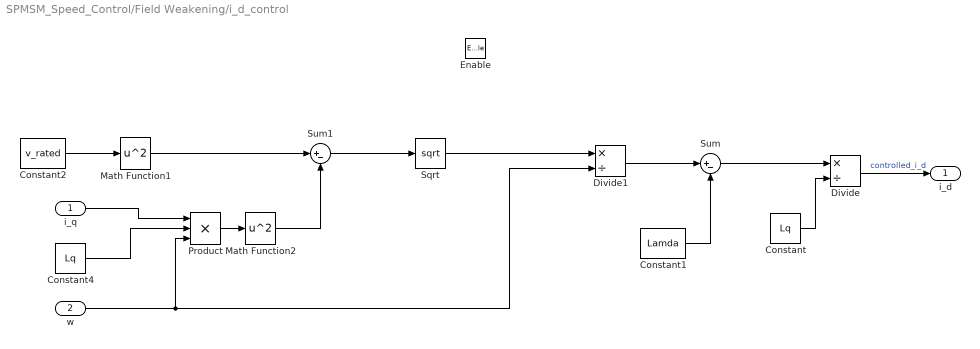
== system SPMSM_Speed_Control/Field Weakening/i_d_control ==
  i_q : Inport
  w : Inport  Port=2
  Enable : EnablePort
  Constant : Constant  Value=Lq
  Constant1 : Constant  Value=Lamda
  Constant2 : Constant  Value=v_rated
  Constant4 : Constant  Value=Lq
  Divide : Product  Inputs=*/
  Divide1 : Product  Inputs=*/
  Math Function1 : Math  Operator=square
  Math Function2 : Math  Operator=square
  Product : Product  Inputs=3
  Sqrt : Sqrt
  Sum : Sum  Inputs=|+-
  Sum1 : Sum  Inputs=|+-
  i_d : Outport
  wires:
  Divide/1 -> i_d/1  "controlled_i_d"
  Constant/1 -> Divide/2
  Sum/1 -> Divide/1
  Constant1/1 -> Sum/2
  Divide1/1 -> Sum/1
  w/1 -> Product/3, Divide1/2
  Sqrt/1 -> Divide1/1
  Sum1/1 -> Sqrt/1
  Constant2/1 -> Math Function1/1
  Math Function1/1 -> Sum1/1
  Product/1 -> Math Function2/1
  Math Function2/1 -> Sum1/2
  Constant4/1 -> Product/2
  i_q/1 -> Product/1

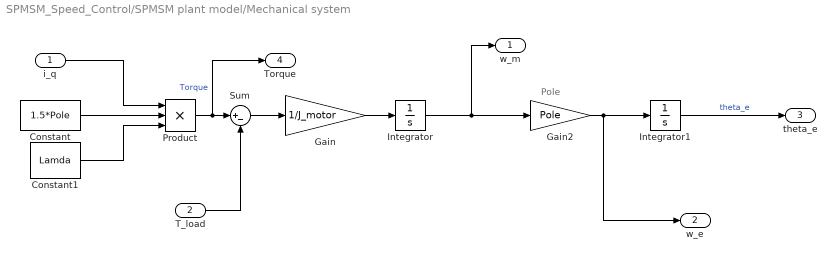
== system SPMSM_Speed_Control/SPMSM plant model/Mechanical system ==
  note: Pole
  i_q : Inport
  T_load : Inport  Port=2
  Constant : Constant  Value=1.5*Pole
  Constant1 : Constant  Value=Lamda
  Gain : Gain  Gain=1/J_motor
  Gain2 : Gain  Gain=Pole
  Integrator : Integrator
  Integrator1 : Integrator
  Product : Product  Inputs=***
  Sum : Sum  Inputs=|+-
  w_m : Outport
  w_e : Outport  Port=2
  theta_e : Outport  Port=3
  Torque : Outport  Port=4
  wires:
  Product/1 -> Torque/1, Sum/1  "Torque"
  Gain2/1 -> w_e/1, Integrator1/1
  Constant1/1 -> Product/3
  Constant/1 -> Product/2
  Integrator/1 -> Gain2/1, w_m/1
  Sum/1 -> Gain/1
  Integrator1/1 -> theta_e/1  "theta_e"
  Gain/1 -> Integrator/1
  i_q/1 -> Product/1
  T_load/1 -> Sum/2

== system SPMSM_Speed_Control/SPMSM plant model/abc2dq ==
  v_abc : Inport
  theta_e : Inport  Port=2
  *sqrt(2/3) : Gain  Gain=sqrt(2/3)  Multiplication=Matrix(K*u)
  Clark Transform : Subsystem
  Demux : Demux  Outputs=2
  Demux1 : Demux  Outputs=3
  Park Transform : Subsystem
  Sine-Cosine Lookup4 : mcbcontrolslib/Sine-Cosine Lookup  AngleInput=Radians  N_points=1024
      settings: LibrarySourceBlock=mcblib/Controls/Math Transforms/Sine-Cosine Lookup
  v_d : Outport
  v_q : Outport  Port=2
  wires:
  v_abc/1 -> *sqrt(2/3)/1
  Demux1/1 -> Clark Transform/1(v_a)
  Demux1/2 -> Clark Transform/2(v_b)
  Demux1/3 -> Clark Transform/3(v_c)
  *sqrt(2/3)/1 -> Demux1/1
  Clark Transform/1(v_xy) -> Park Transform/1(v_xy)  "v_xy"
  Park Transform/1(v_dq) -> Demux/1
  Demux/1 -> v_d/1  "v_d"
  Demux/2 -> v_q/1  "v_q"
  Sine-Cosine Lookup4/1 -> Park Transform/2(sin_theta)  "sin"
  theta_e/1 -> Sine-Cosine Lookup4/1
  Sine-Cosine Lookup4/2 -> Park Transform/3(cos_theta)  "cos"

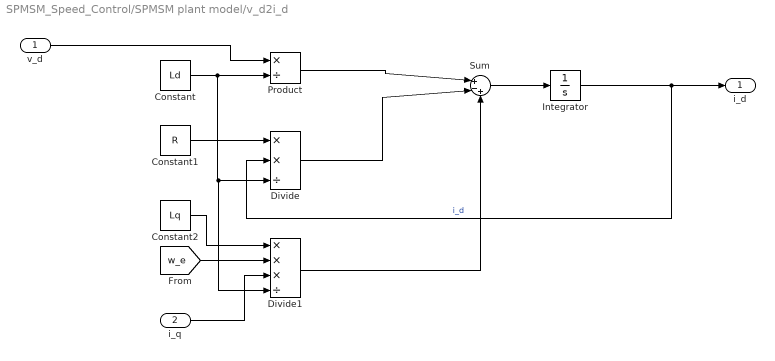
== system SPMSM_Speed_Control/SPMSM plant model/v_d2i_d ==
  v_d : Inport
  i_q : Inport  Port=2
  Constant : Constant  Value=Ld
  Constant1 : Constant  Value=R
  Constant2 : Constant  Value=Lq
  Divide : Product  Inputs=**/
  Divide1 : Product  Inputs=***/
  Integrator : Integrator
  Product : Product  Inputs=*/
  Sum : Sum  Inputs=|+-+
  i_d : Outport
  wires:
  Sum/1 -> Integrator/1
  Divide/1 -> Sum/2
  [w_e] -> Divide1/2
  Constant2/1 -> Divide1/1
  Integrator/1 -> i_d/1, Divide/2  "i_d"
  Constant/1 -> Divide1/4, Divide/3, Product/2
  Divide1/1 -> Sum/3
  i_q/1 -> Divide1/3
  Constant1/1 -> Divide/1
  Product/1 -> Sum/1
  v_d/1 -> Product/1

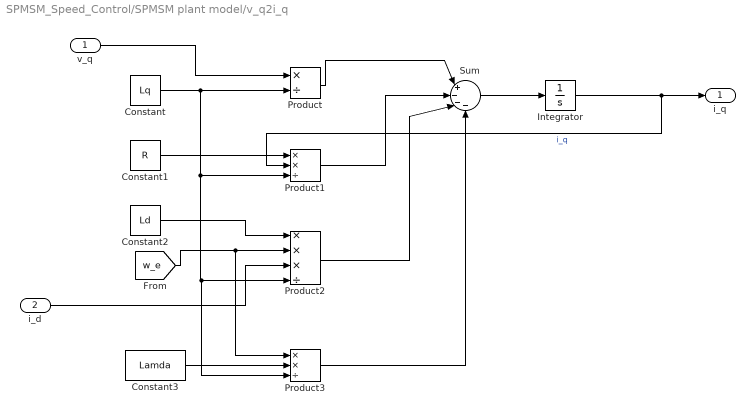
== system SPMSM_Speed_Control/SPMSM plant model/v_q2i_q ==
  v_q : Inport
  i_d : Inport  Port=2
  Constant : Constant  Value=Lq
  Constant1 : Constant  Value=R
  Constant2 : Constant  Value=Ld
  Constant3 : Constant  Value=Lamda
  Integrator : Integrator
  Product : Product  Inputs=*/
  Product1 : Product  Inputs=**/
  Product2 : Product  Inputs=***/
  Product3 : Product  Inputs=**/
  Sum : Sum  Inputs=|+---
  i_q : Outport
  wires:
  Integrator/1 -> i_q/1, Product1/2  "i_q"
  Sum/1 -> Integrator/1
  v_q/1 -> Product/1
  Constant/1 -> Product3/3, Product2/4, Product1/3, Product/2
  Product/1 -> Sum/1
  Constant1/1 -> Product1/1
  Product1/1 -> Sum/2
  Constant2/1 -> Product2/1
  [w_e] -> Product3/1, Product2/2
  i_d/1 -> Product2/3
  Product2/1 -> Sum/3
  Product3/1 -> Sum/4
  Constant3/1 -> Product3/2

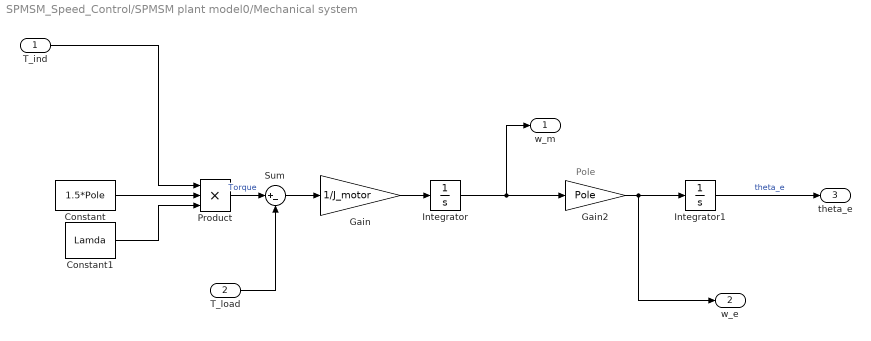
== system SPMSM_Speed_Control/SPMSM plant model0/Mechanical system ==
  note: Pole
  T_ind : Inport
  T_load : Inport  Port=2
  Constant : Constant  Value=1.5*Pole
  Constant1 : Constant  Value=Lamda
  Gain : Gain  Gain=1/J_motor
  Gain2 : Gain  Gain=Pole
  Integrator : Integrator
  Integrator1 : Integrator
  Product : Product  Inputs=***
  Sum : Sum  Inputs=|+-
  w_m : Outport
  w_e : Outport  Port=2
  theta_e : Outport  Port=3
  wires:
  Product/1 -> Sum/1  "Torque"
  Gain2/1 -> w_e/1, Integrator1/1
  Constant1/1 -> Product/3
  Constant/1 -> Product/2
  Integrator/1 -> Gain2/1, w_m/1
  Sum/1 -> Gain/1
  Integrator1/1 -> theta_e/1  "theta_e"
  Gain/1 -> Integrator/1
  T_ind/1 -> Product/1
  T_load/1 -> Sum/2

== system SPMSM_Speed_Control/SPMSM plant model0/abc2dq ==
  v_abc : Inport
  theta_e : Inport  Port=2
  *sqrt(2/3) : Gain  Gain=sqrt(2/3)  Multiplication=Matrix(K*u)
  Clark Transform : Subsystem
  Demux : Demux  Outputs=2
  Demux1 : Demux  Outputs=3
  Park Transform : Subsystem
  Sine-Cosine Lookup4 : mcbcontrolslib/Sine-Cosine Lookup  AngleInput=Radians  N_points=1024
      settings: LibrarySourceBlock=mcblib/Controls/Math Transforms/Sine-Cosine Lookup
  v_d : Outport
  v_q : Outport  Port=2
  wires:
  v_abc/1 -> *sqrt(2/3)/1  "v_abc"
  Demux1/1 -> Clark Transform/1(v_a)
  Demux1/2 -> Clark Transform/2(v_b)
  Demux1/3 -> Clark Transform/3(v_c)
  *sqrt(2/3)/1 -> Demux1/1
  Clark Transform/1(v_xy) -> Park Transform/1(v_xy)  "v_xy"
  Park Transform/1(v_dq) -> Demux/1
  Demux/1 -> v_d/1  "v_d"
  Demux/2 -> v_q/1  "v_q"
  Sine-Cosine Lookup4/1 -> Park Transform/2(sin_theta)  "ssin"
  theta_e/1 -> Sine-Cosine Lookup4/1
  Sine-Cosine Lookup4/2 -> Park Transform/3(cos_theta)  "ccos"

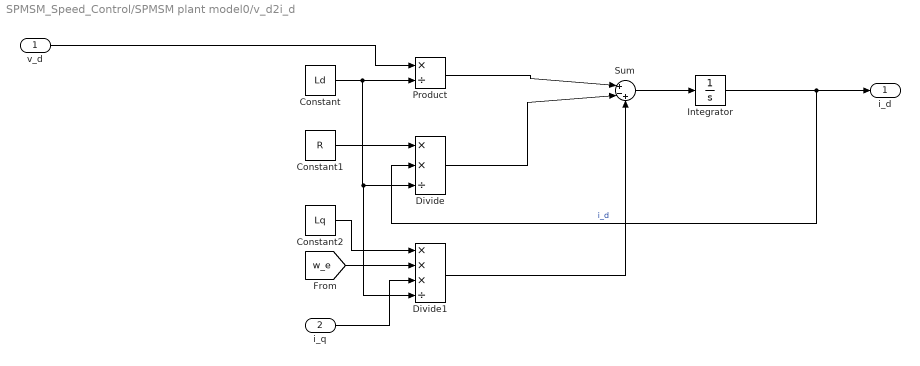
== system SPMSM_Speed_Control/SPMSM plant model0/v_d2i_d ==
  v_d : Inport
  i_q : Inport  Port=2
  Constant : Constant  Value=Ld
  Constant1 : Constant  Value=R
  Constant2 : Constant  Value=Lq
  Divide : Product  Inputs=**/
  Divide1 : Product  Inputs=***/
  Integrator : Integrator
  Product : Product  Inputs=*/
  Sum : Sum  Inputs=|+-+
  i_d : Outport
  wires:
  Sum/1 -> Integrator/1
  Divide/1 -> Sum/2
  [w_e] -> Divide1/2
  Constant2/1 -> Divide1/1
  Integrator/1 -> i_d/1, Divide/2  "i_d"
  Constant/1 -> Divide1/4, Divide/3, Product/2
  Divide1/1 -> Sum/3
  i_q/1 -> Divide1/3
  Constant1/1 -> Divide/1
  Product/1 -> Sum/1
  v_d/1 -> Product/1

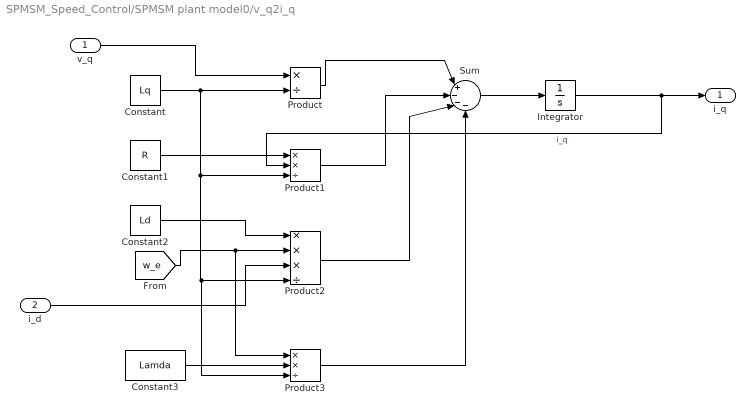
== system SPMSM_Speed_Control/SPMSM plant model0/v_q2i_q ==
  v_q : Inport
  i_d : Inport  Port=2
  Constant : Constant  Value=Lq
  Constant1 : Constant  Value=R
  Constant2 : Constant  Value=Ld
  Constant3 : Constant  Value=Lamda
  Integrator : Integrator
  Product : Product  Inputs=*/
  Product1 : Product  Inputs=**/
  Product2 : Product  Inputs=***/
  Product3 : Product  Inputs=**/
  Sum : Sum  Inputs=|+---
  i_q : Outport
  wires:
  Integrator/1 -> i_q/1, Product1/2  "i_q"
  Sum/1 -> Integrator/1
  v_q/1 -> Product/1
  Constant/1 -> Product3/3, Product2/4, Product1/3, Product/2
  Product/1 -> Sum/1
  Constant1/1 -> Product1/1
  Product1/1 -> Sum/2
  Constant2/1 -> Product2/1
  [w_e] -> Product3/1, Product2/2
  i_d/1 -> Product2/3
  Product2/1 -> Sum/3
  Product3/1 -> Sum/4
  Constant3/1 -> Product3/2

== system SPMSM_Speed_Control/dq2abc/dq2xy ==
  v_d : Inport
  v_q : Inport  Port=2
  sin_theta : Inport  Port=3
  cos_theta : Inport  Port=4
  Mux : Mux  Inputs=2
  Product{,1..3} (4 alike) : Product
  Sum : Sum  Inputs=|+-
  Sum1 : Sum  Inputs=|++
  v_xy : Outport
  wires:
  v_d/1 -> Product2/1, Product/1
  cos_theta/1 -> Product/2, Product3/2
  v_q/1 -> Product3/1, Product1/1
  sin_theta/1 -> Product2/2, Product1/2
  Product/1 -> Sum/1
  Product1/1 -> Sum/2
  Sum/1 -> Mux/1  "v_x"
  Product2/1 -> Sum1/1
  Product3/1 -> Sum1/2
  Sum1/1 -> Mux/2  "v_y"
  Mux/1 -> v_xy/1

== system SPMSM_Speed_Control/dq2abc/xy2abc ==
  v_xy : Inport
  Demux : Demux  Outputs=2
  Gain1 : Gain  Gain=-1/2
  Gain2 : Gain  Gain=sqrt(3)/2
  Gain3 : Gain  Gain=-1/2
  Gain4 : Gain  Gain=-sqrt(3)/2
  Sum : Sum  Inputs=|++
  Sum1 : Sum  Inputs=|++
  v_a : Outport
  v_b : Outport  Port=2
  v_c : Outport  Port=3
  wires:
  v_xy/1 -> Demux/1
  Demux/1 -> Gain3/1, Gain1/1, v_a/1  "v_x"
  Demux/2 -> Gain4/1, Gain2/1  "v_y"
  Sum/1 -> v_b/1
  Gain1/1 -> Sum/1
  Gain2/1 -> Sum/2
  Sum1/1 -> v_c/1
  Gain4/1 -> Sum1/2
  Gain3/1 -> Sum1/1

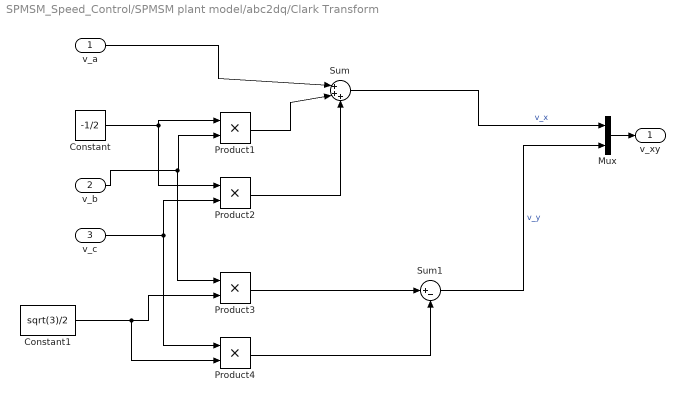
== system SPMSM_Speed_Control/SPMSM plant model/abc2dq/Clark Transform ==
  v_a : Inport
  v_b : Inport  Port=2
  v_c : Inport  Port=3
  Constant : Constant  Value=-1/2
  Constant1 : Constant  Value=sqrt(3)/2
  Mux : Mux  Inputs=2
  Product{1..4} (4 alike) : Product
  Sum : Sum  Inputs=|+++
  Sum1 : Sum  Inputs=|+-
  v_xy : Outport
  wires:
  v_a/1 -> Sum/1
  Constant/1 -> Product1/1, Product2/1
  v_b/1 -> Product3/1, Product1/2
  Product1/1 -> Sum/2
  v_c/1 -> Product4/1, Product2/2
  Product2/1 -> Sum/3
  Constant1/1 -> Product4/2, Product3/2
  Product3/1 -> Sum1/1
  Product4/1 -> Sum1/2
  Mux/1 -> v_xy/1
  Sum/1 -> Mux/1  "v_x"
  Sum1/1 -> Mux/2  "v_y"

== system SPMSM_Speed_Control/SPMSM plant model/abc2dq/Park Transform ==
  v_xy : Inport
  sin_theta : Inport  Port=2
  cos_theta : Inport  Port=3
  Demux : Demux  Outputs=2
  Mux : Mux  Inputs=2
  Product{,1..3} (4 alike) : Product
  Sum : Sum  Inputs=|++
  Sum1 : Sum  Inputs=|-+
  v_dq : Outport
  wires:
  v_xy/1 -> Demux/1
  Demux/1 -> Product/1, Product2/1  "v_x"
  Demux/2 -> Product3/1, Product1/1  "v_y"
  cos_theta/1 -> Product3/2, Product/2
  sin_theta/1 -> Product2/2, Product1/2
  Product/1 -> Sum/1
  Product1/1 -> Sum/2
  Sum/1 -> Mux/1  "v_d"
  Product2/1 -> Sum1/1
  Product3/1 -> Sum1/2
  Sum1/1 -> Mux/2  "v_q"
  Mux/1 -> v_dq/1  "v_dq"

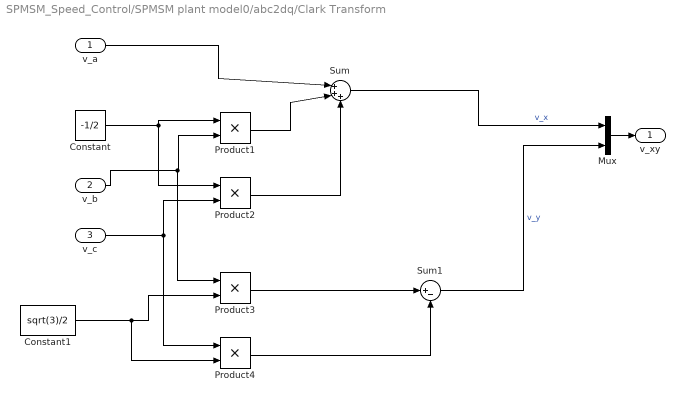
== system SPMSM_Speed_Control/SPMSM plant model0/abc2dq/Clark Transform ==
  v_a : Inport
  v_b : Inport  Port=2
  v_c : Inport  Port=3
  Constant : Constant  Value=-1/2
  Constant1 : Constant  Value=sqrt(3)/2
  Mux : Mux  Inputs=2
  Product{1..4} (4 alike) : Product
  Sum : Sum  Inputs=|+++
  Sum1 : Sum  Inputs=|+-
  v_xy : Outport
  wires:
  v_a/1 -> Sum/1
  Constant/1 -> Product1/1, Product2/1
  v_b/1 -> Product3/1, Product1/2
  Product1/1 -> Sum/2
  v_c/1 -> Product4/1, Product2/2
  Product2/1 -> Sum/3
  Constant1/1 -> Product4/2, Product3/2
  Product3/1 -> Sum1/1
  Product4/1 -> Sum1/2
  Mux/1 -> v_xy/1
  Sum/1 -> Mux/1  "v_x"
  Sum1/1 -> Mux/2  "v_y"

== system SPMSM_Speed_Control/SPMSM plant model0/abc2dq/Park Transform ==
  v_xy : Inport
  sin_theta : Inport  Port=2
  cos_theta : Inport  Port=3
  Demux : Demux  Outputs=2
  Mux : Mux  Inputs=2
  Product{,1..3} (4 alike) : Product
  Sum : Sum  Inputs=|++
  Sum1 : Sum  Inputs=|-+
  v_dq : Outport
  wires:
  v_xy/1 -> Demux/1
  Demux/1 -> Product/1, Product2/1  "v_x"
  Demux/2 -> Product3/1, Product1/1  "v_y"
  cos_theta/1 -> Product3/2, Product/2
  sin_theta/1 -> Product2/2, Product1/2
  Product/1 -> Sum/1
  Product1/1 -> Sum/2
  Sum/1 -> Mux/1  "v_d"
  Product2/1 -> Sum1/1
  Product3/1 -> Sum1/2
  Sum1/1 -> Mux/2  "v_q"
  Mux/1 -> v_dq/1  "v_dq"
